simulink model "gm_uz_sine_generator_16bit"  (R2023a)
settings: Solver=FixedStepDiscrete  StartTime=0.0  StopTime=50000/100e6  RelTol=1e-3
libraries: hdlsllib x8, embmathops x8, simulink x1
(part 2 of 2)

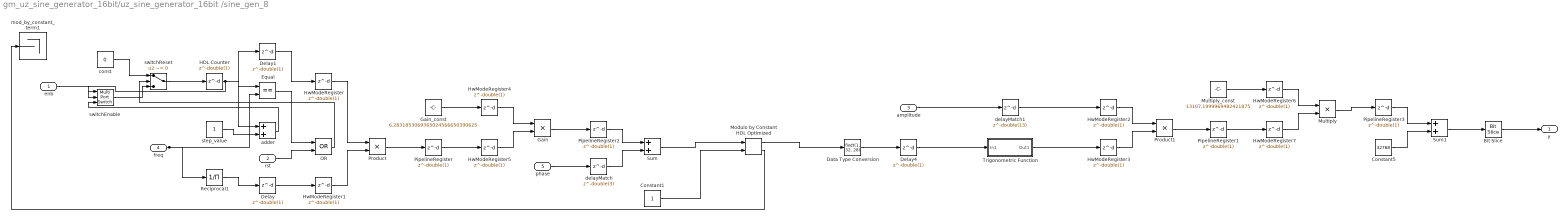
== system gm_uz_sine_generator_16bit/uz_sine_generator_16bit /sine_gen_8 ==
  enb : Inport  OutDataTypeStr=boolean  PortDimensions=1  SampleTime=1e-08
  rst : Inport  Port=2  OutDataTypeStr=boolean  PortDimensions=1  SampleTime=1e-08
  amplitude : Inport  Port=3  OutDataTypeStr=fixdt(1, 32, 28)  PortDimensions=1  SampleTime=1e-08
  freq : Inport  Port=4  OutDataTypeStr=uint32  PortDimensions=1  SampleTime=1e-08
  phase : Inport  Port=5  OutDataTypeStr=fixdt(1, 16, 12)  PortDimensions=1  SampleTime=1e-08
  Bit Slice : hdlsllib/Logic and Bit Operations/Bit Slice  lidx=double(15)  ridx=double(0)
  Constant1 : Constant  OutDataTypeStr=boolean  SampleTime=1e-08
  Constant5 : Constant  Value=32768  OutDataTypeStr=int32  SampleTime=1e-08
  Data Type Conversion : DataTypeConversion  OutDataTypeStr=fixdt(1, 32, 28)  SampleTime=1e-08  SaturateOnIntegerOverflow=off  RndMeth=Floor
  Delay : Delay  DelayLength=double(1)  InitialCondition=0  SampleTime=1e-08
  Delay1 : Delay  DelayLength=double(1)  InitialCondition=0  SampleTime=1e-08
  Delay4 : Delay  DelayLength=double(1)  InitialCondition=0  SampleTime=1e-08
  Equal : RelationalOperator  Operator===  OutDataTypeStr=boolean  SampleTime=1e-08  InputSameDT=off
  Gain : Product  Inputs=**  OutDataTypeStr=fixdt(1, 32, 28)  SampleTime=1e-08
  Gain_const : Constant  Value=6.2831853069365024566650390625  OutDataTypeStr=fixdt(0, 32, 29)  SampleTime=1e-08
  HDL Counter : Delay  DelayLength=double(1)  InitialCondition=0  SampleTime=1e-08
  HwModeRegister{,1..7} (8 alike) : Delay  DelayLength=double(1)  InitialCondition=0  SampleTime=1e-08
  Modulo by Constant HDL Optimized : embmathops/Modulo by Constant HDL Optimized  Denominator=2*pi  SimulateUsing=Code generation
      settings: LibrarySourceBlock=|
      | embeddedMatrixLib/Math Operations/Modulo by Constant
      | HDL Optimized
  Multiply : Product  Inputs=**  OutDataTypeStr=int32  SampleTime=1e-08
  Multiply_const : Constant  Value=13107.1999969482421875  OutDataTypeStr=fixdt(1, 32, 17)  SampleTime=1e-08
  OR : Logic  Operator=OR  AllPortsSameDT=off  OutDataTypeStr=boolean  SampleTime=1e-08
  PipelineRegister{,1..3} (4 alike) : Delay  DelayLength=double(1)  InitialCondition=0  SampleTime=1e-08
  Product : Product  Inputs=**  OutDataTypeStr=fixdt(0, 32, 29)  SampleTime=1e-08
  Product1 : Product  Inputs=**  OutDataTypeStr=fixdt(1, 32, 28)  SampleTime=1e-08
  Reciprocal1 : Product  Inputs=/  OutDataTypeStr=fixdt(0, 32, 31)  RndMeth=Zero  SaturateOnIntegerOverflow=on  SampleTime=1e-08
  Sum : Sum  AccumDataTypeStr=fixdt(1, 33, 28)  OutDataTypeStr=fixdt(1, 33, 28)  SampleTime=1e-08
  Sum1 : Sum  AccumDataTypeStr=int32  OutDataTypeStr=int32  SampleTime=1e-08
  Trigonometric Function : Subsystem
  adder : Sum  AccumDataTypeStr=uint32  OutDataTypeStr=uint32  SampleTime=1e-08
  const : Constant  Value=0  VectorParams1D=off  OutDataTypeStr=uint32  SampleTime=1e-08
  delayMatch : Delay  DelayLength=double(3)  InitialCondition=0  SampleTime=1e-08
  delayMatch1 : Delay  DelayLength=double(13)  InitialCondition=0  SampleTime=1e-08
  mod_by_constant_term1 : Terminator
  step_value : Constant  VectorParams1D=off  OutDataTypeStr=uint32  SampleTime=1e-08
  switchEnable : MultiPortSwitch  DataPortOrder=Zero-based contiguous  Inputs=2  DiagnosticForDefault=None  zeroidx=on  OutDataTypeStr=uint32  SampleTime=1e-08  SaturateOnIntegerOverflow=off  InputSameDT=off
  switchReset : Switch  Criteria=u2 ~= 0  Threshold=double(0)  OutDataTypeStr=uint32  SampleTime=1e-08  SaturateOnIntegerOverflow=off  InputSameDT=off
  y : Outport  SampleTime=1e-08
  wires:
  delayMatch1/1 -> HwModeRegister2/1
  delayMatch/1 -> Sum/2
  Bit Slice/1 -> y/1
  Constant1/1 -> Modulo by Constant HDL Optimized/2
  Constant5/1 -> Sum1/2
  Data Type Conversion/1 -> Delay4/1
  Delay/1 -> HwModeRegister1/1
  Delay1/1 -> HwModeRegister/1
  Sum/1 -> Modulo by Constant HDL Optimized/1
  Delay4/1 -> Trigonometric Function/1(In1)
  Trigonometric Function/1(Out1) -> HwModeRegister3/1
  PipelineRegister2/1 -> Sum/1
  Modulo by Constant HDL Optimized/1 -> Data Type Conversion/1
  Modulo by Constant HDL Optimized/2 -> mod_by_constant_term1/1
  PipelineRegister3/1 -> Sum1/1
  PipelineRegister/1 -> HwModeRegister5/1
  PipelineRegister1/1 -> HwModeRegister7/1
  Reciprocal1/1 -> Delay/1
  Sum1/1 -> Bit Slice/1
  HDL Counter/1 -> Delay1/1, Equal/1, adder/1, switchEnable/2
  const/1 -> switchReset/1
  step_value/1 -> adder/2
  Gain_const/1 -> HwModeRegister4/1
  Multiply_const/1 -> HwModeRegister6/1
  enb/1 -> switchEnable/1
  rst/1 -> OR/2
  amplitude/1 -> delayMatch1/1
  freq/1 -> Reciprocal1/1, Equal/2
  phase/1 -> delayMatch/1
  switchReset/1 -> HDL Counter/1
  adder/1 -> switchEnable/3
  switchEnable/1 -> switchReset/3
  Equal/1 -> OR/1
  OR/1 -> switchReset/2
  Product/1 -> PipelineRegister/1
  HwModeRegister/1 -> Product/1
  HwModeRegister1/1 -> Product/2
  Product1/1 -> PipelineRegister1/1
  HwModeRegister2/1 -> Product1/1
  HwModeRegister3/1 -> Product1/2
  Gain/1 -> PipelineRegister2/1
  HwModeRegister4/1 -> Gain/1
  HwModeRegister5/1 -> Gain/2
  Multiply/1 -> PipelineRegister3/1
  HwModeRegister6/1 -> Multiply/1
  HwModeRegister7/1 -> Multiply/2

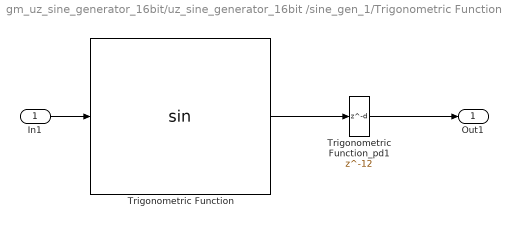
== system gm_uz_sine_generator_16bit/uz_sine_generator_16bit /sine_gen_1/Trigonometric Function ==
  In1 : Inport
  Trigonometric Function : Trigonometry  ApproximationMethod=CORDIC
  Trigonometric Function_pd1 : Delay  DelayLength=12
  Out1 : Outport
  wires:
  Trigonometric Function_pd1/1 -> Out1/1
  Trigonometric Function/1 -> Trigonometric Function_pd1/1
  In1/1 -> Trigonometric Function/1

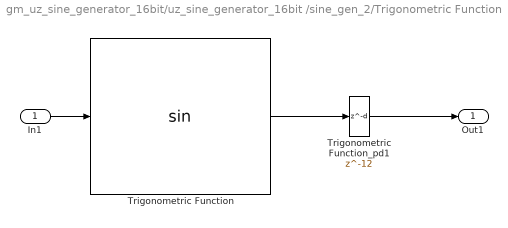
== system gm_uz_sine_generator_16bit/uz_sine_generator_16bit /sine_gen_2/Trigonometric Function ==
  In1 : Inport
  Trigonometric Function : Trigonometry  ApproximationMethod=CORDIC
  Trigonometric Function_pd1 : Delay  DelayLength=12
  Out1 : Outport
  wires:
  Trigonometric Function_pd1/1 -> Out1/1
  Trigonometric Function/1 -> Trigonometric Function_pd1/1
  In1/1 -> Trigonometric Function/1

== system gm_uz_sine_generator_16bit/uz_sine_generator_16bit /sine_gen_3/Trigonometric Function ==
  In1 : Inport
  Trigonometric Function : Trigonometry  ApproximationMethod=CORDIC
  Trigonometric Function_pd1 : Delay  DelayLength=12
  Out1 : Outport
  wires:
  Trigonometric Function_pd1/1 -> Out1/1
  Trigonometric Function/1 -> Trigonometric Function_pd1/1
  In1/1 -> Trigonometric Function/1

== system gm_uz_sine_generator_16bit/uz_sine_generator_16bit /sine_gen_4/Trigonometric Function ==
  In1 : Inport
  Trigonometric Function : Trigonometry  ApproximationMethod=CORDIC
  Trigonometric Function_pd1 : Delay  DelayLength=12
  Out1 : Outport
  wires:
  Trigonometric Function_pd1/1 -> Out1/1
  Trigonometric Function/1 -> Trigonometric Function_pd1/1
  In1/1 -> Trigonometric Function/1

== system gm_uz_sine_generator_16bit/uz_sine_generator_16bit /sine_gen_5/Trigonometric Function ==
  In1 : Inport
  Trigonometric Function : Trigonometry  ApproximationMethod=CORDIC
  Trigonometric Function_pd1 : Delay  DelayLength=12
  Out1 : Outport
  wires:
  Trigonometric Function_pd1/1 -> Out1/1
  Trigonometric Function/1 -> Trigonometric Function_pd1/1
  In1/1 -> Trigonometric Function/1

== system gm_uz_sine_generator_16bit/uz_sine_generator_16bit /sine_gen_6/Trigonometric Function ==
  In1 : Inport
  Trigonometric Function : Trigonometry  ApproximationMethod=CORDIC
  Trigonometric Function_pd1 : Delay  DelayLength=12
  Out1 : Outport
  wires:
  Trigonometric Function_pd1/1 -> Out1/1
  Trigonometric Function/1 -> Trigonometric Function_pd1/1
  In1/1 -> Trigonometric Function/1

== system gm_uz_sine_generator_16bit/uz_sine_generator_16bit /sine_gen_7/Trigonometric Function ==
  In1 : Inport
  Trigonometric Function : Trigonometry  ApproximationMethod=CORDIC
  Trigonometric Function_pd1 : Delay  DelayLength=12
  Out1 : Outport
  wires:
  Trigonometric Function_pd1/1 -> Out1/1
  Trigonometric Function/1 -> Trigonometric Function_pd1/1
  In1/1 -> Trigonometric Function/1

== system gm_uz_sine_generator_16bit/uz_sine_generator_16bit /sine_gen_8/Trigonometric Function ==
  In1 : Inport
  Trigonometric Function : Trigonometry  ApproximationMethod=CORDIC
  Trigonometric Function_pd1 : Delay  DelayLength=12
  Out1 : Outport
  wires:
  Trigonometric Function/1 -> Trigonometric Function_pd1/1
  Trigonometric Function_pd1/1 -> Out1/1
  In1/1 -> Trigonometric Function/1
